simulink model "controller_Harness_PedalPosition"  (R2023b)
settings: Solver=FixedStepAuto  StartTime=0.0  StopTime=13  FixedStep=1/100  RelTol=1e-3
libraries: simulink x2
settings Model: Creator=Matteo  LastModifiedBy=dadog
settings OptimizationCC: ReuseModelBlockBuffer=off
settings DebuggingCC: UnconnectedInputMsg=warning  UnconnectedOutputMsg=warning  UnconnectedLineMsg=warning
settings ModelReferenceCC: EnableRefExpFcnMdlSchedulingChecks=on
settings RTWCC: DLArmComputeVersion=19.05
settings ConfigComp: CovEnable=on  CovScope=Subsystem  RecordCoverage=on  CovSaveSingleToWorkspaceVar=on

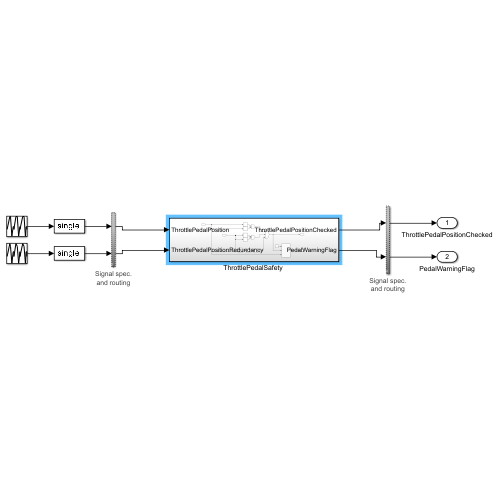
[thumbnail: Simulink's stored preview of the top-level diagram]
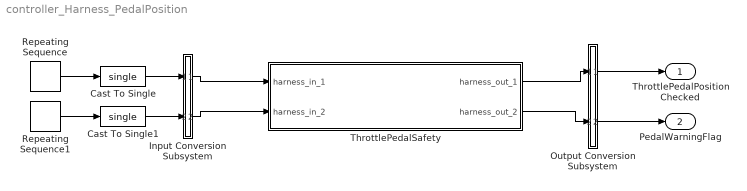
== system controller_Harness_PedalPosition ==
  Cast To Single : DataTypeConversion  OutDataTypeStr=single  SaturateOnIntegerOverflow=off  RndMeth=Floor
  Cast To Single1 : DataTypeConversion  OutDataTypeStr=single  SaturateOnIntegerOverflow=off  RndMeth=Floor
  Input Conversion Subsystem : Subsystem  Tag=__SLT_ICS__  Description=|
      | Signal spec.
      | and routing
      settings: AttributesFormatString=%<Description>
  Output Conversion Subsystem : Subsystem  Tag=__SLT_OCS__  Description=|
      | Signal spec.
      | and routing
      settings: AttributesFormatString=%<Description>
  Repeating Sequence : simulink/Sources/Repeating Sequence  rep_seq_t=[0 5 7 10 12 13]  rep_seq_y=[0 1 1 -0.5 0.2 0.2]
  Repeating Sequence1 : simulink/Sources/Repeating Sequence  rep_seq_t=[0 5 7 10 12 13]  rep_seq_y=[0 1 0.8 -0.5 0.4 0.4]
  "ThrottlePedalSafety " : Subsystem  Tag=__SL_testing_harness_stub_
  ThrottlePedalPositionChecked : Outport
  PedalWarningFlag : Outport  Port=2
  wires:
  Repeating Sequence/1 -> Cast To Single/1
  Repeating Sequence1/1 -> Cast To Single1/1
  Output Conversion Subsystem/1(Outport_1) -> ThrottlePedalPositionChecked/1
  Output Conversion Subsystem/2(Outport_2) -> PedalWarningFlag/1
  Input Conversion Subsystem/1(Outport_1) -> "ThrottlePedalSafety "/1(harness_in_1)
  Input Conversion Subsystem/2(Outport_2) -> "ThrottlePedalSafety "/2(harness_in_2)
  "ThrottlePedalSafety "/1(harness_out_1) -> Output Conversion Subsystem/1(Inport_1)
  "ThrottlePedalSafety "/2(harness_out_2) -> Output Conversion Subsystem/2(Inport_2)
  Cast To Single/1 -> Input Conversion Subsystem/1(Inport_1)
  Cast To Single1/1 -> Input Conversion Subsystem/2(Inport_2)

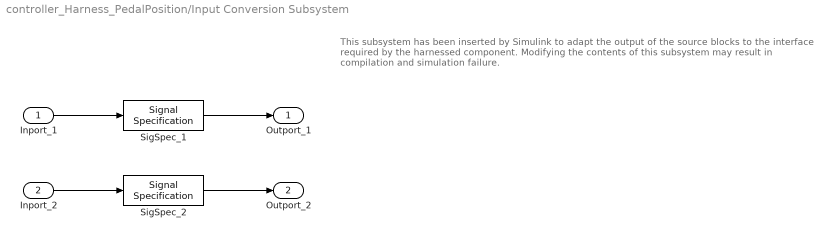
== system controller_Harness_PedalPosition/Input Conversion Subsystem ==
  note: This subsystem has been inserted by Simulink to adapt the output of the source blocks to the interface required by the harnessed component.
      |  Modifying the contents of this subsystem may result in compilation and simulation failure.
  Inport_1 : Inport
  Inport_2 : Inport  Port=2
  SigSpec_1 : SignalSpecification  OutDataTypeStr=single  Dimensions=[1]  SampleTime=0.01
  SigSpec_2 : SignalSpecification  OutDataTypeStr=single  Dimensions=[1]  SampleTime=0.01
  Outport_1 : Outport
  Outport_2 : Outport  Port=2
  wires:
  SigSpec_1/1 -> Outport_1/1
  Inport_1/1 -> SigSpec_1/1
  SigSpec_2/1 -> Outport_2/1
  Inport_2/1 -> SigSpec_2/1

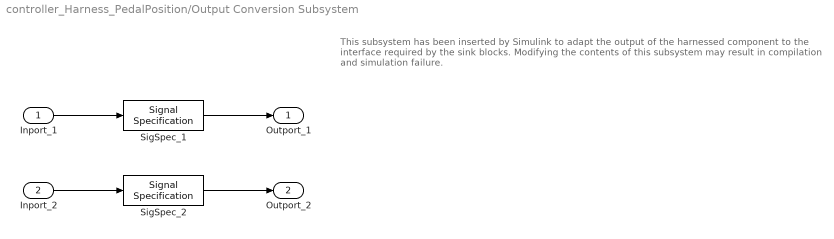
== system controller_Harness_PedalPosition/Output Conversion Subsystem ==
  note: This subsystem has been inserted by Simulink to adapt the output of the harnessed component to the interface required by the sink blocks.
      |  Modifying the contents of this subsystem may result in compilation and simulation failure.
  Inport_1 : Inport
  Inport_2 : Inport  Port=2
  SigSpec_1 : SignalSpecification  OutDataTypeStr=single  Dimensions=[1]  SampleTime=0.01
  SigSpec_2 : SignalSpecification  OutDataTypeStr=boolean  Dimensions=[1]  SampleTime=0.01
  Outport_1 : Outport
  Outport_2 : Outport  Port=2
  wires:
  Inport_1/1 -> SigSpec_1/1
  SigSpec_1/1 -> Outport_1/1
  Inport_2/1 -> SigSpec_2/1
  SigSpec_2/1 -> Outport_2/1

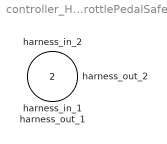
== system controller_Harness_PedalPosition/ThrottlePedalSafety  ==
  harness_in_1 : Inport
  harness_in_2 : Inport  Port=2
  harness_out_1 : Outport
  harness_out_2 : Outport  Port=2
